simulink model "sampleModel1753_5_sub"  (R2023a)
settings: Solver=VariableStepAuto  StartTime=0.0  StopTime=10.0  RelTol=1e-3
libraries: hdlsllib x4, simulink x1
settings Model: Creator=user1  LastModifiedBy=user1

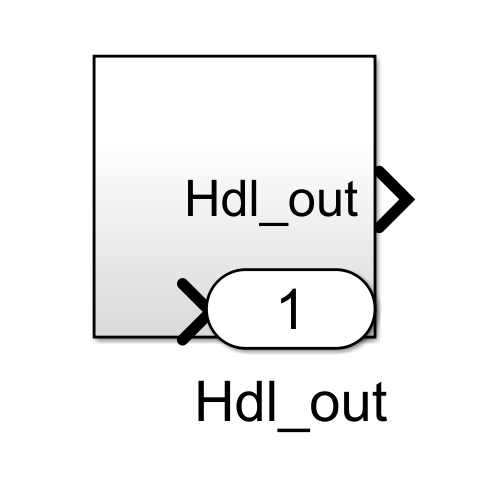
[thumbnail: Simulink's stored preview of the top-level diagram]
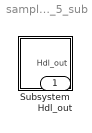
== system sampleModel1753_5_sub ==
  Subsystem : Subsystem
  Hdl_out : Outport  OutDataTypeStr=uint8

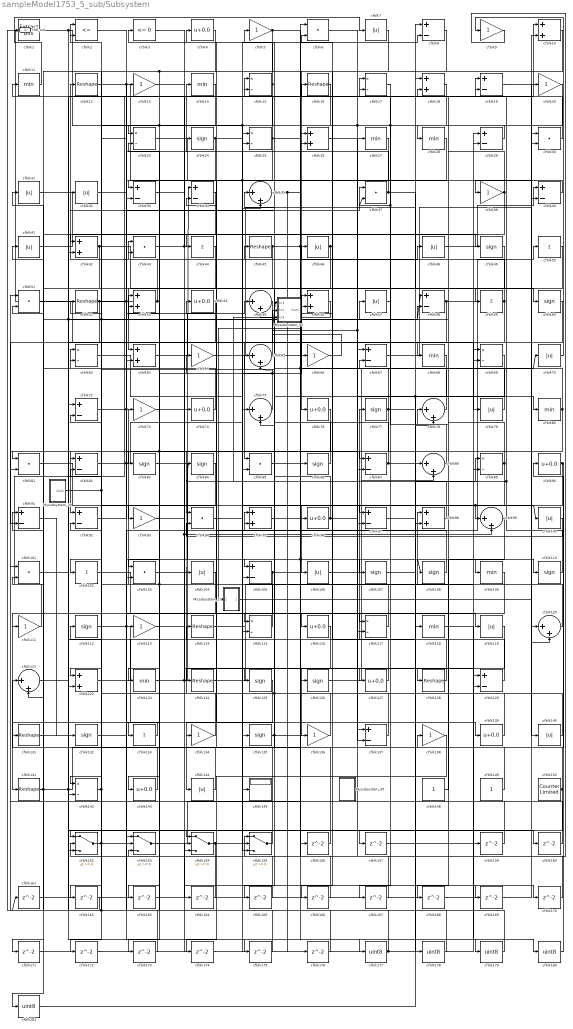
== system sampleModel1753_5_sub/Subsystem ==
  Mysubsystem_17 : Subsystem  TreatAsAtomicUnit=on  RTWFcnName=Mysubsystem_17
      settings: RTWFcnNameOpts=User specified  RTWFileNameOpts=Use function name
  Mysubsystem_29 : Subsystem  TreatAsAtomicUnit=on  RTWFcnName=Mysubsystem_29
      settings: RTWFcnNameOpts=User specified  RTWFileNameOpts=Use function name
  Mysubsystem_32 : Subsystem  TreatAsAtomicUnit=on  RTWFcnName=Mysubsystem_32
      settings: RTWFcnNameOpts=User specified  RTWFileNameOpts=Use function name
  Mysubsystem_45 : Subsystem  TreatAsAtomicUnit=on  RTWFcnName=Mysubsystem_45
      settings: RTWFcnNameOpts=User specified  RTWFileNameOpts=Use function name
  cfblk1 : simulink/Logic and Bit Operations/Extract Bits  bitsToExtract=Upper half  numBits=8  bitIdxRange=[0 7]  outScalingMode=Preserve fixed-point scaling
      settings: LibrarySourceBlock=|
      | hdlsllib/Logic and Bit
      | Operations/Extract Bits
  cfblk{10,18,26,42,53,56,63,95,98,122} (10 alike) : Sum  OutDataTypeStr=uint8
  cfblk{7,31..32,41,46,48,57,70,79,100,104,106,119,140,144} (15 alike) : Abs  OutDataTypeStr=uint8  SaturateOnIntegerOverflow=off
  cfblk{6,30,37,43,51,81,85,94,101,103} (10 alike) : DotProduct  OutDataTypeStr=uint8
  cfblk{44,50,59,102,133} (5 alike) : Sum  Inputs=+  OutDataTypeStr=uint8
  cfblk{8,19,29,33..34,40,58,67,72,82,87,91..92,97,105,129,137} (17 alike) : Sum  Inputs=+-  OutDataTypeStr=uint8
  cfblk{24,49,60,77,83..84,86,107..108,110,112,125..126,132,135} (15 alike) : Signum
  cfblk{11,14,27..28,68,80,109,118,123} (9 alike) : MinMax  OutDataTypeStr=uint8
  cfblk{5,9,13,20,39,64,66,73,93,111,113,134,136,138} (14 alike) : Gain  OutDataTypeStr=uint8
  cfblk{12,16,45,52,114,124,128,131,141} (9 alike) : Reshape
  cfblk{15,17,23,25,62,69,89,115,117,142} (10 alike) : Product  Inputs=*/  OutDataTypeStr=uint8  RndMeth=Zero  SaturateOnIntegerOverflow=on
  cfblk{4,54,74,76,90,96,116,127,139,143} (10 alike) : Bias  Bias=0.0  SaturateOnIntegerOverflow=off
  cfblk{35,55,65,75,78,88,99,120..121} (9 alike) : Sum  Inputs=|++  OutDataTypeStr=uint8
  cfblk145 : Display
  cfblk148 : Constant  OutDataTypeStr=uint8  SampleTime=-1
  cfblk149 : Constant  OutDataTypeStr=uint8  SampleTime=-1
  cfblk150 : hdlsllib/Sources/Counter Limited  uplimit=7  tsamp=-1
  cfblk{152..155} (4 alike) : Switch  OutDataTypeStr=uint8  SaturateOnIntegerOverflow=off  InputSameDT=off
  cfblk{156..157,159..176} (20 alike) : Delay  SampleTime=1
  cfblk{177..181} (5 alike) : DataTypeConversion  OutDataTypeStr=uint8  SaturateOnIntegerOverflow=off  RndMeth=Floor
  cfblk2 : RelationalOperator  Operator=<=  OutDataTypeStr=boolean  InputSameDT=off
  cfblk3 : hdlsllib/Logic and Bit Operations/Compare To Zero  relop=<=  OutDataTypeStr=uint8
  Hdl_out : Outport  OutDataTypeStr=uint8
  wires:
  cfblk15/1 -> cfblk3/1, cfblk33/2, cfblk155/2
  cfblk28/1 -> cfblk33/1
  cfblk65/1 -> cfblk170/1, cfblk2/1, cfblk41/1
  cfblk91/1 -> cfblk132/1
  cfblk112/1 -> cfblk139/1
  cfblk120/1 -> cfblk73/1
  cfblk137/1 -> cfblk65/2, cfblk34/1
  cfblk125/1 -> cfblk144/1
  cfblk89/1 -> cfblk53/2, cfblk106/1
  cfblk82/1 -> cfblk160/1, cfblk66/1
  cfblk83/1 -> cfblk105/1
  cfblk111/1 -> cfblk10/1
  cfblk77/1 -> cfblk78/2, cfblk32/1, cfblk94/1
  cfblk155/1 -> cfblk4/1
  cfblk7/1 -> cfblk76/1
  cfblk126/1 -> cfblk88/2
  cfblk48/1 -> cfblk40/1
  cfblk68/1 -> cfblk166/1, cfblk98/2
  cfblk50/1 -> cfblk93/1
  cfblk136/1 -> cfblk43/1
  cfblk10/1 -> cfblk96/1
  cfblk123/1 -> cfblk58/2, cfblk27/1
  cfblk19/1 -> cfblk120/1
  cfblk103/1 -> cfblk50/1
  cfblk109/1 -> cfblk141/1
  cfblk59/1 -> cfblk2/2, cfblk127/1
  cfblk76/1 -> cfblk92/1
  cfblk2/1 -> cfblk109/1
  cfblk70/1 -> cfblk9/1
  cfblk12/1 -> cfblk87/2, cfblk137/1
  cfblk124/1 -> cfblk69/1
  cfblk52/1 -> cfblk91/2, cfblk137/2, cfblk13/1
  cfblk39/1 -> cfblk42/2, cfblk28/1
  cfblk114/1 -> cfblk98/1
  cfblk40/1 -> cfblk39/1
  cfblk25/1 -> cfblk123/1, cfblk19/2, cfblk11/1
  cfblk106/1 -> cfblk29/1
  cfblk27/1 -> cfblk134/1
  cfblk81/1 -> cfblk140/1
  cfblk110/1 -> cfblk15/2, cfblk84/1
  cfblk60/1 -> cfblk115/1
  cfblk23/1 -> cfblk135/1
  cfblk87/1 -> cfblk64/1, cfblk100/1, cfblk99/1
  cfblk108/1 -> cfblk34/2
  cfblk34/1 -> cfblk111/1
  cfblk72/1 -> cfblk37/1, cfblk119/1
  cfblk94/1 -> cfblk145/1
  cfblk1/1 -> cfblk69/2, cfblk25/2
  cfblk127/1 -> cfblk46/1
  cfblk140/1 -> cfblk62/1
  cfblk119/1 -> cfblk136/1
  cfblk142/1 -> cfblk162/1, cfblk62/2
  cfblk115/1 -> cfblk54/1
  cfblk41/1 -> cfblk44/1
  cfblk116/1 -> cfblk124/1
  cfblk153/1 -> cfblk126/1
  cfblk3/1 -> cfblk105/2, cfblk99/2
  cfblk11/1 -> cfblk7/1
  cfblk135/1 -> cfblk35/1, cfblk70/1, cfblk48/1
  cfblk16/1 -> cfblk102/1
  cfblk67/1 -> cfblk30/1
  cfblk24/1 -> cfblk153/2, cfblk40/2, cfblk128/1
  cfblk46/1 -> cfblk63/1, cfblk116/1
  cfblk102/1 -> cfblk115/2
  cfblk144/1 -> cfblk51/2
  cfblk53/1 -> Hdl_out/1, cfblk83/1, cfblk12/1
  cfblk84/1 -> cfblk122/1
  cfblk79/1 -> cfblk6/2
  cfblk8/1 -> cfblk42/1
  cfblk64/1 -> cfblk8/1
  cfblk55/1 -> cfblk85/1
  cfblk131/1 -> cfblk154/1
  cfblk90/1 -> cfblk155/3, cfblk138/1
  cfblk113/1 -> cfblk74/1
  cfblk42/1 -> cfblk121/2, cfblk60/1
  cfblk86/1 -> cfblk15/1
  cfblk29/1 -> cfblk23/1
  cfblk152/1 -> cfblk72/2, cfblk95/2, cfblk113/1
  cfblk141/1 -> cfblk181/1, cfblk91/1, cfblk86/1, cfblk17/2, cfblk58/1
  cfblk121/1 -> cfblk114/1
  cfblk117/1 -> cfblk43/2, cfblk92/2
  cfblk51/1 -> cfblk79/1
  cfblk129/1 -> cfblk77/1
  cfblk30/1 -> cfblk5/1
  cfblk122/1 -> cfblk18/1
  cfblk44/1 -> cfblk103/1
  cfblk5/1 -> cfblk63/2, cfblk107/1
  cfblk4/1 -> cfblk143/1, cfblk81/1
  cfblk75/1 -> cfblk53/1, cfblk52/1
  cfblk139/1 -> cfblk18/2
  cfblk54/1 -> cfblk103/2
  cfblk20/1 -> cfblk117/2, cfblk173/1, cfblk172/1
  cfblk92/1 -> cfblk55/1
  cfblk9/1 -> cfblk155/1
  cfblk96/1 -> cfblk110/1, cfblk45/1
  cfblk58/1 -> cfblk171/1, cfblk20/1
  cfblk69/1 -> cfblk75/2
  cfblk101/1 -> cfblk177/1
  cfblk74/1 -> cfblk31/1
  cfblk143/1 -> cfblk121/1
  cfblk104/1 -> cfblk142/1
  cfblk149/1 -> cfblk65/1
  cfblk37/1 -> cfblk59/1, cfblk14/1
  cfblk88/1 -> cfblk67/2
  cfblk31/1 -> cfblk97/2, Mysubsystem_32/1(In1)
  cfblk56/1 -> cfblk55/2
  cfblk63/1 -> cfblk8/2
  cfblk78/1 -> cfblk56/1
  cfblk154/1 -> cfblk152/2, cfblk57/1
  cfblk80/1 -> cfblk37/2, cfblk17/1, cfblk133/1, cfblk81/2
  cfblk133/1 -> cfblk131/1
  cfblk32/1 -> cfblk24/1
  cfblk128/1 -> cfblk56/2
  cfblk150/1 -> cfblk152/3, cfblk95/1
  cfblk6/1 -> cfblk129/2
  cfblk45/1 -> cfblk122/2, cfblk68/1, cfblk49/1
  cfblk26/1 -> cfblk80/1
  cfblk93/1 -> cfblk97/1
  cfblk18/1 -> cfblk167/1, cfblk82/1
  cfblk35/1 -> cfblk176/1, cfblk26/2
  cfblk100/1 -> cfblk94/2
  cfblk95/1 -> cfblk179/1, cfblk108/1
  cfblk134/1 -> cfblk112/1
  cfblk73/1 -> cfblk125/1
  cfblk62/1 -> cfblk85/2
  cfblk148/1 -> cfblk78/1
  cfblk107/1 -> cfblk89/1
  cfblk43/1 -> cfblk16/1, cfblk104/1
  cfblk17/1 -> cfblk87/1
  cfblk105/1 -> cfblk142/2, cfblk117/1
  cfblk85/1 -> cfblk156/1
  cfblk156/1 -> cfblk25/1
  cfblk57/1 -> cfblk157/1
  cfblk157/1 -> cfblk89/2
  cfblk159/1 -> cfblk129/1
  cfblk160/1 -> cfblk51/1
  cfblk161/1 -> cfblk29/2
  cfblk162/1 -> cfblk1/1
  cfblk14/1 -> cfblk163/1
  cfblk163/1 -> cfblk35/2
  cfblk13/1 -> cfblk164/1
  cfblk164/1 -> cfblk154/2
  cfblk49/1 -> cfblk165/1
  cfblk165/1 -> cfblk23/2
  cfblk166/1 -> cfblk6/1
  cfblk167/1 -> cfblk26/1
  cfblk99/1 -> cfblk168/1
  cfblk168/1 -> cfblk10/2
  cfblk33/1 -> cfblk169/1
  cfblk169/1 -> cfblk120/2
  cfblk170/1 -> cfblk67/1
  cfblk171/1 -> cfblk154/3
  cfblk172/1 -> cfblk75/1
  cfblk173/1 -> cfblk72/1
  cfblk138/1 -> cfblk174/1
  cfblk174/1 -> cfblk88/1
  cfblk132/1 -> cfblk175/1
  cfblk175/1 -> cfblk153/1
  cfblk176/1 -> cfblk153/3
  cfblk177/1 -> cfblk159/1, cfblk82/2, cfblk161/1
  cfblk97/1 -> cfblk178/1
  cfblk178/1 -> cfblk101/1
  cfblk179/1 -> cfblk101/2
  cfblk118/1 -> cfblk180/1
  cfblk180/1 -> cfblk90/1
  cfblk181/1 -> cfblk118/1
  Mysubsystem_17/1(Out1) -> cfblk30/2
  Mysubsystem_29/1(Out1) -> cfblk152/1, cfblk19/1
  cfblk66/1 -> Mysubsystem_32/2(In2)
  cfblk98/1 -> Mysubsystem_32/3(In3)
  Mysubsystem_32/1(Out1) -> Mysubsystem_17/1(In1)

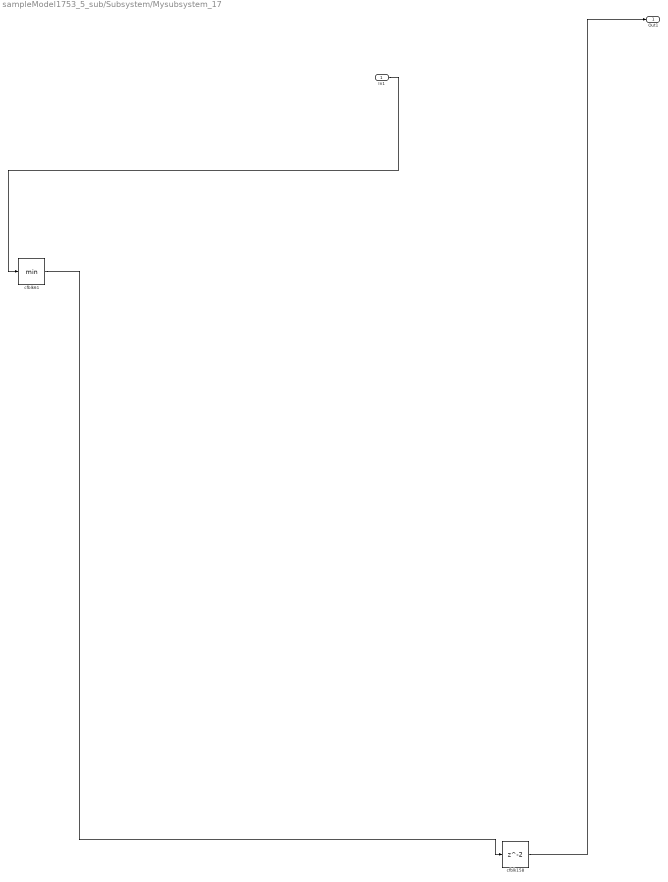
== system sampleModel1753_5_sub/Subsystem/Mysubsystem_17 ==
  In1 : Inport
  cfblk158 : Delay  SampleTime=1
  cfblk61 : MinMax
  Out1 : Outport
  wires:
  In1/1 -> cfblk61/1
  cfblk158/1 -> Out1/1
  cfblk61/1 -> cfblk158/1

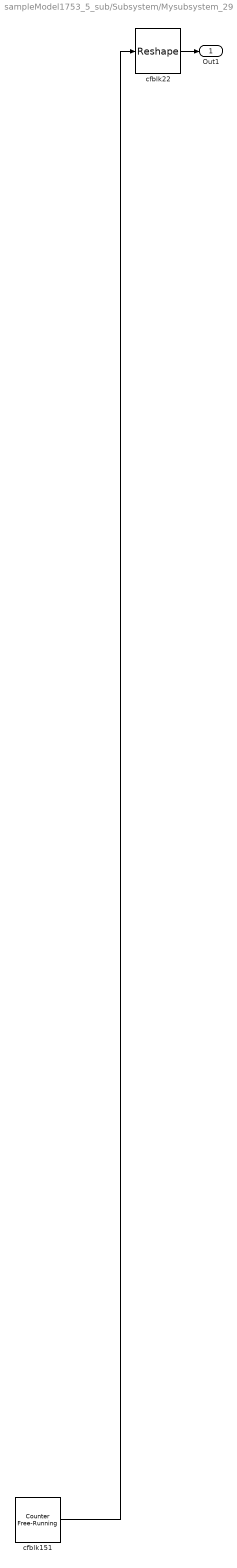
== system sampleModel1753_5_sub/Subsystem/Mysubsystem_29 ==
  cfblk151 : hdlsllib/Sources/Counter Free-Running  NumBits=16  tsamp=-1
  cfblk22 : Reshape
  Out1 : Outport
  wires:
  cfblk22/1 -> Out1/1
  cfblk151/1 -> cfblk22/1

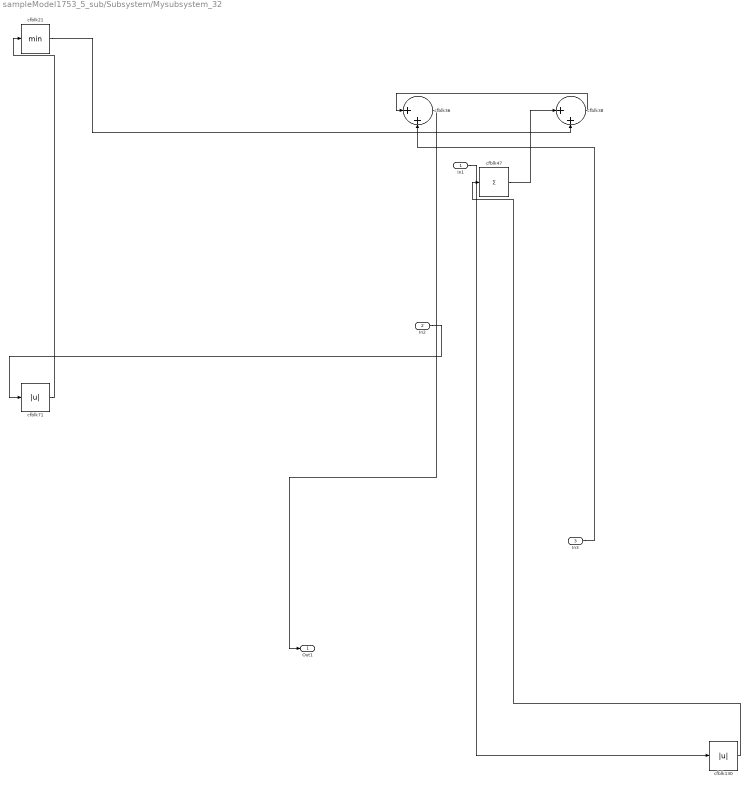
== system sampleModel1753_5_sub/Subsystem/Mysubsystem_32 ==
  In1 : Inport
  In2 : Inport  Port=2
  In3 : Inport  Port=3
  cfblk130 : Abs  SaturateOnIntegerOverflow=off
  cfblk21 : MinMax
  cfblk36 : Sum  Inputs=|++
  cfblk38 : Sum  Inputs=|++
  cfblk47 : Sum  Inputs=+
  cfblk71 : Abs  SaturateOnIntegerOverflow=off
  Out1 : Outport
  wires:
  In1/1 -> cfblk130/1
  cfblk38/1 -> cfblk36/1
  In3/1 -> cfblk36/2
  cfblk130/1 -> cfblk47/1
  cfblk36/1 -> Out1/1
  In2/1 -> cfblk71/1
  cfblk71/1 -> cfblk21/1
  cfblk21/1 -> cfblk38/2
  cfblk47/1 -> cfblk38/1

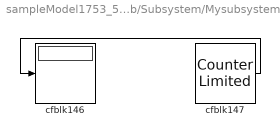
== system sampleModel1753_5_sub/Subsystem/Mysubsystem_45 ==
  cfblk146 : Display
  cfblk147 : hdlsllib/Sources/Counter Limited  uplimit=7  tsamp=-1
  wires:
  cfblk147/1 -> cfblk146/1
